simulink library "LkpTbl_Lib"  (Simulink 7.7)
settings: Solver=ode45  StartTime=0.0  StopTime=10.0  RelTol=1e-3
settings Model: Creator=jzqwf2  LastModifiedBy=MT22BENCH

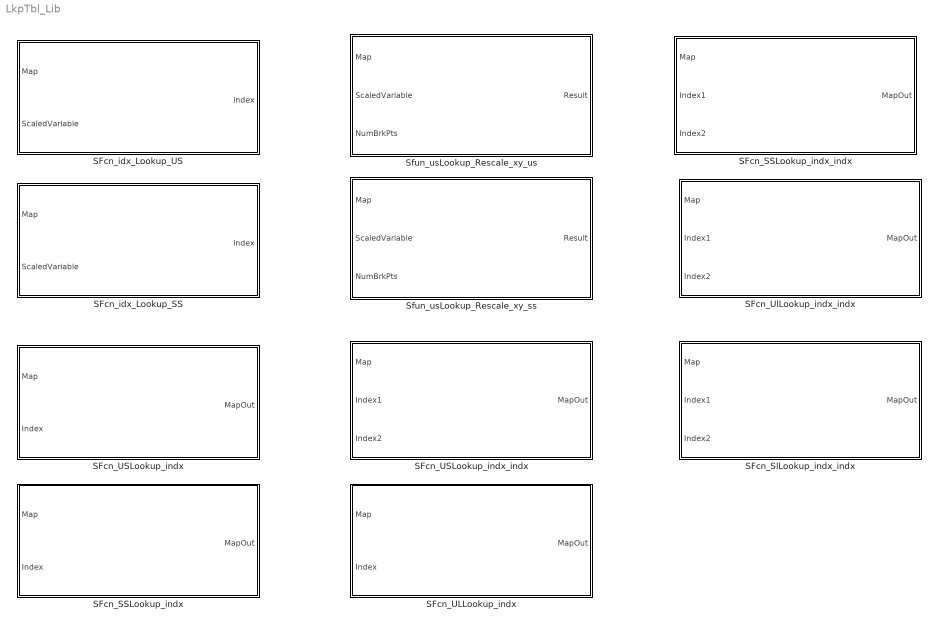
== system LkpTbl_Lib ==
  SFcn_SSLookup_indx : Subsystem  TreatAsAtomicUnit=on
      settings: RTWSystemCode=Inline
  SFcn_SSLookup_indx_indx : Subsystem  TreatAsAtomicUnit=on
      settings: RTWSystemCode=Inline
  SFcn_SlLookup_indx_indx : Subsystem  TreatAsAtomicUnit=on
      settings: RTWSystemCode=Inline
  SFcn_ULLookup_indx : Subsystem  TreatAsAtomicUnit=on
      settings: RTWSystemCode=Inline
  SFcn_USLookup_indx : Subsystem  TreatAsAtomicUnit=on
      settings: RTWSystemCode=Inline
  SFcn_USLookup_indx_indx : Subsystem  TreatAsAtomicUnit=on
      settings: RTWSystemCode=Inline
  SFcn_UlLookup_indx_indx : Subsystem  TreatAsAtomicUnit=on
      settings: RTWSystemCode=Inline
  SFcn_idx_Lookup_SS : Subsystem  TreatAsAtomicUnit=on
      settings: RTWSystemCode=Inline
  SFcn_idx_Lookup_US : Subsystem  TreatAsAtomicUnit=on
      settings: RTWSystemCode=Inline
  Sfun_usLookup_Rescale_xy_ss : Subsystem  TreatAsAtomicUnit=on
      settings: RTWSystemCode=Inline
  Sfun_usLookup_Rescale_xy_us : Subsystem  TreatAsAtomicUnit=on
      settings: RTWSystemCode=Inline

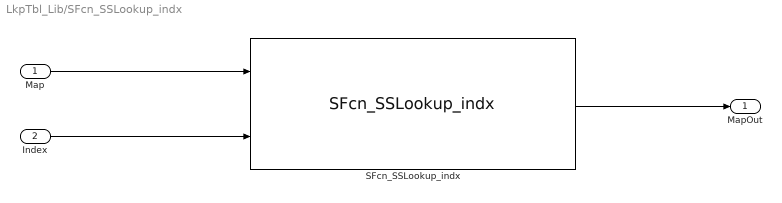
== system LkpTbl_Lib/SFcn_SSLookup_indx ==
  Map : Inport
  Index : Inport  Port=2
  SFcn_SSLookup_indx : S-Function  FunctionName=SFcn_SSLookup_indx  EnableBusSupport=off
  MapOut : Outport
  wires:
  SFcn_SSLookup_indx/1 -> MapOut/1
  Index/1 -> SFcn_SSLookup_indx/2
  Map/1 -> SFcn_SSLookup_indx/1

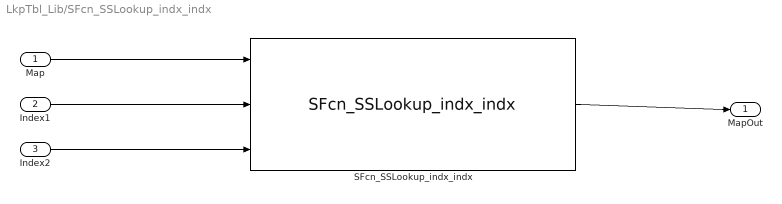
== system LkpTbl_Lib/SFcn_SSLookup_indx_indx ==
  Map : Inport
  Index1 : Inport  Port=2
  Index2 : Inport  Port=3
  SFcn_SSLookup_indx_indx : S-Function  FunctionName=SFcn_SSLookup_indx_indx  EnableBusSupport=off
  MapOut : Outport
  wires:
  Index2/1 -> SFcn_SSLookup_indx_indx/3
  SFcn_SSLookup_indx_indx/1 -> MapOut/1
  Index1/1 -> SFcn_SSLookup_indx_indx/2
  Map/1 -> SFcn_SSLookup_indx_indx/1

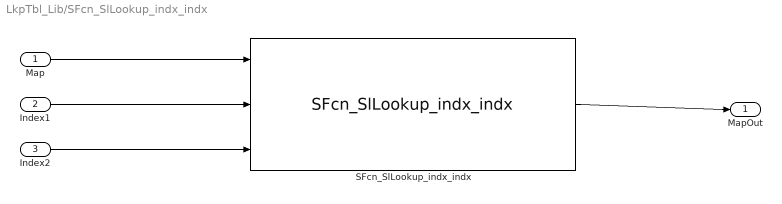
== system LkpTbl_Lib/SFcn_SlLookup_indx_indx ==
  Map : Inport
  Index1 : Inport  Port=2
  Index2 : Inport  Port=3
  SFcn_SlLookup_indx_indx : S-Function  FunctionName=SFcn_SlLookup_indx_indx  EnableBusSupport=off
  MapOut : Outport
  wires:
  Map/1 -> SFcn_SlLookup_indx_indx/1
  Index1/1 -> SFcn_SlLookup_indx_indx/2
  SFcn_SlLookup_indx_indx/1 -> MapOut/1
  Index2/1 -> SFcn_SlLookup_indx_indx/3

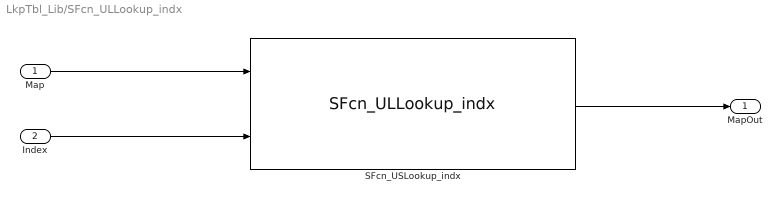
== system LkpTbl_Lib/SFcn_ULLookup_indx ==
  Map : Inport
  Index : Inport  Port=2
  SFcn_USLookup_indx : S-Function  FunctionName=SFcn_ULLookup_indx  EnableBusSupport=off
  MapOut : Outport
  wires:
  SFcn_USLookup_indx/1 -> MapOut/1
  Index/1 -> SFcn_USLookup_indx/2
  Map/1 -> SFcn_USLookup_indx/1

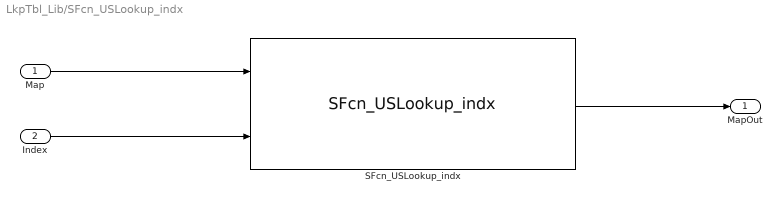
== system LkpTbl_Lib/SFcn_USLookup_indx ==
  Map : Inport
  Index : Inport  Port=2
  SFcn_USLookup_indx : S-Function  FunctionName=SFcn_USLookup_indx  EnableBusSupport=off
  MapOut : Outport
  wires:
  Map/1 -> SFcn_USLookup_indx/1
  Index/1 -> SFcn_USLookup_indx/2
  SFcn_USLookup_indx/1 -> MapOut/1

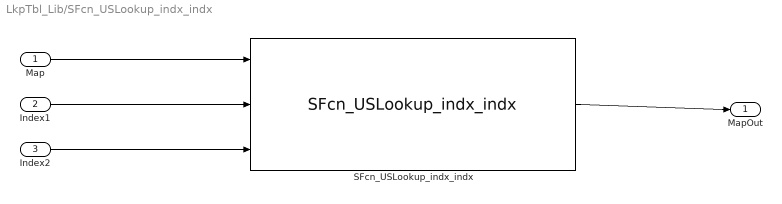
== system LkpTbl_Lib/SFcn_USLookup_indx_indx ==
  Map : Inport
  Index1 : Inport  Port=2
  Index2 : Inport  Port=3
  SFcn_USLookup_indx_indx : S-Function  FunctionName=SFcn_USLookup_indx_indx  EnableBusSupport=off
  MapOut : Outport
  wires:
  Map/1 -> SFcn_USLookup_indx_indx/1
  Index1/1 -> SFcn_USLookup_indx_indx/2
  SFcn_USLookup_indx_indx/1 -> MapOut/1
  Index2/1 -> SFcn_USLookup_indx_indx/3

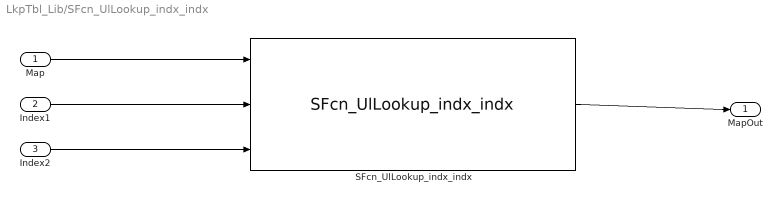
== system LkpTbl_Lib/SFcn_UlLookup_indx_indx ==
  Map : Inport
  Index1 : Inport  Port=2
  Index2 : Inport  Port=3
  SFcn_UlLookup_indx_indx : S-Function  FunctionName=SFcn_UlLookup_indx_indx  EnableBusSupport=off
  MapOut : Outport
  wires:
  Index2/1 -> SFcn_UlLookup_indx_indx/3
  SFcn_UlLookup_indx_indx/1 -> MapOut/1
  Index1/1 -> SFcn_UlLookup_indx_indx/2
  Map/1 -> SFcn_UlLookup_indx_indx/1

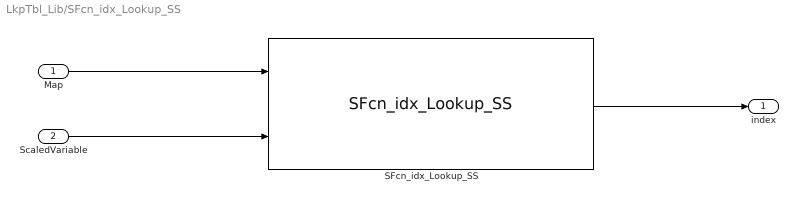
== system LkpTbl_Lib/SFcn_idx_Lookup_SS ==
  Map : Inport
  ScaledVariable : Inport  Port=2
  SFcn_idx_Lookup_SS : S-Function  FunctionName=SFcn_idx_Lookup_SS  EnableBusSupport=off
  index : Outport
  wires:
  SFcn_idx_Lookup_SS/1 -> index/1
  ScaledVariable/1 -> SFcn_idx_Lookup_SS/2
  Map/1 -> SFcn_idx_Lookup_SS/1

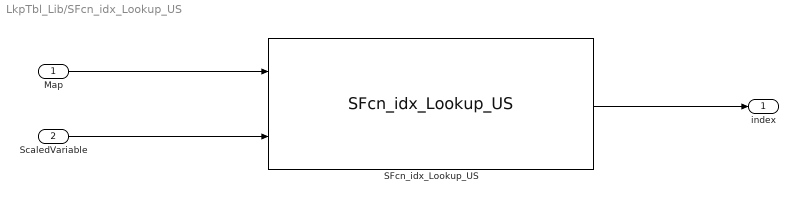
== system LkpTbl_Lib/SFcn_idx_Lookup_US ==
  Map : Inport
  ScaledVariable : Inport  Port=2
  SFcn_idx_Lookup_US : S-Function  FunctionName=SFcn_idx_Lookup_US  EnableBusSupport=off
  index : Outport
  wires:
  Map/1 -> SFcn_idx_Lookup_US/1
  ScaledVariable/1 -> SFcn_idx_Lookup_US/2
  SFcn_idx_Lookup_US/1 -> index/1

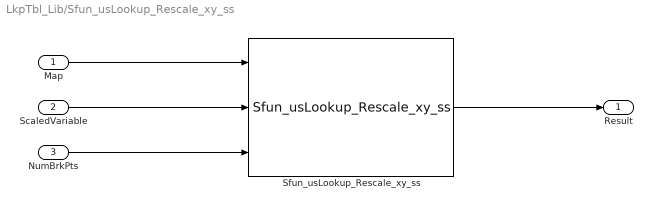
== system LkpTbl_Lib/Sfun_usLookup_Rescale_xy_ss ==
  Map : Inport
  ScaledVariable : Inport  Port=2
  NumBrkPts : Inport  Port=3
  Sfun_usLookup_Rescale_xy_ss : S-Function  FunctionName=Sfun_usLookup_Rescale_xy_ss  EnableBusSupport=off
  Result : Outport
  wires:
  Sfun_usLookup_Rescale_xy_ss/1 -> Result/1
  NumBrkPts/1 -> Sfun_usLookup_Rescale_xy_ss/3
  ScaledVariable/1 -> Sfun_usLookup_Rescale_xy_ss/2
  Map/1 -> Sfun_usLookup_Rescale_xy_ss/1

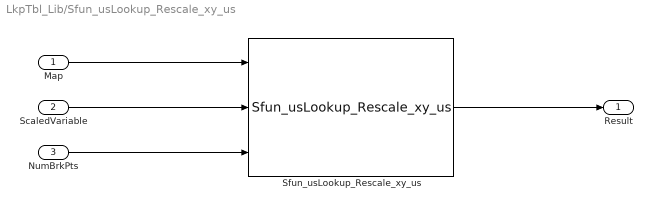
== system LkpTbl_Lib/Sfun_usLookup_Rescale_xy_us ==
  Map : Inport
  ScaledVariable : Inport  Port=2
  NumBrkPts : Inport  Port=3
  Sfun_usLookup_Rescale_xy_us : S-Function  FunctionName=Sfun_usLookup_Rescale_xy_us  EnableBusSupport=off
  Result : Outport
  wires:
  NumBrkPts/1 -> Sfun_usLookup_Rescale_xy_us/3
  Map/1 -> Sfun_usLookup_Rescale_xy_us/1
  Sfun_usLookup_Rescale_xy_us/1 -> Result/1
  ScaledVariable/1 -> Sfun_usLookup_Rescale_xy_us/2
